simulink library "iterationReset_ul"  (R2018a)
settings: Solver=VariableStepAuto  StartTime=0.0  StopTime=10.0  RelTol=1e-3
undefined symbols (not defined in the file): simulationPhase_enum
libraries: simulink x2
settings Model: Creator=mitch  LastModifiedBy=mitch

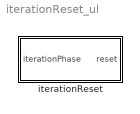
== system iterationReset_ul ==
  iterationReset : Subsystem

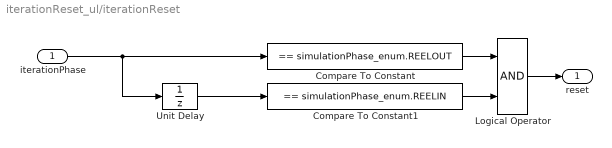
== system iterationReset_ul/iterationReset ==
  iterationPhase : Inport  OutDataTypeStr=Enum: simulationPhase_enum
  Compare To Constant : simulink/Logic and Bit Operations/Compare To Constant  relop===  const=simulationPhase_enum.REELOUT  OutDataTypeStr=boolean
  Compare To Constant1 : simulink/Logic and Bit Operations/Compare To Constant  relop===  const=simulationPhase_enum.REELIN  OutDataTypeStr=boolean
  Logical Operator : Logic  AllPortsSameDT=off  OutDataTypeStr=boolean
  Unit Delay : UnitDelay  SampleTime=-1
  reset : Outport  OutDataTypeStr=boolean
  wires:
  Unit Delay/1 -> Compare To Constant1/1
  iterationPhase/1 -> Unit Delay/1, Compare To Constant/1
  Compare To Constant/1 -> Logical Operator/1
  Compare To Constant1/1 -> Logical Operator/2
  Logical Operator/1 -> reset/1
